simulink model "water_heat"  (R2024b)
settings: Solver=VariableStepAuto  StartTime=0.0  StopTime=10.0  RelTol=1e-3
settings Model: Creator=DELL  LastModifiedBy=DELL

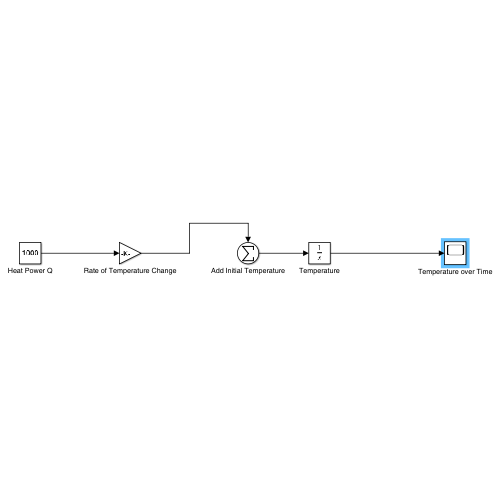
[thumbnail: Simulink's stored preview of the top-level diagram]
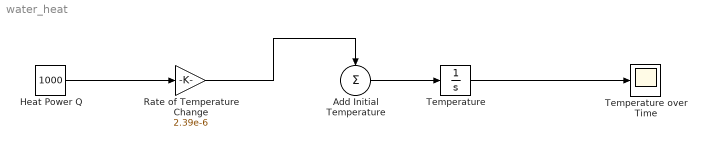
== system water_heat ==
  Add Initial Temperature : Sum  Inputs=+|
  Heat Power Q : Constant  Value=1000
  Rate of Temperature Change : Gain  Gain=2.39e-6
  Temperature : Integrator  InitialCondition=20
  Temperature over Time : Scope
  wires:
  Heat Power Q/1 -> Rate of Temperature Change/1
  Rate of Temperature Change/1 -> Add Initial Temperature/1
  Add Initial Temperature/1 -> Temperature/1
  Temperature/1 -> Temperature over Time/1
